simulink model "bms_controller"  (R2024b)
settings: Solver=FixedStepDiscrete  StartTime=0.0  StopTime=3600  FixedStep=0.1  RelTol=1e-3
undefined symbols (not defined in the file): DiscIntNeverNeededParam
libraries: simulink x6
settings Model: Creator=ferdi  LastModifiedBy=ferdi
settings OptimizationCC: DefaultParameterBehavior=Inlined  EnhancedBackFolding=on  PassReuseOutputArgsAs=Individual arguments  ZeroExternalMemoryAtStartup=off  ZeroInternalMemoryAtStartup=off  OptimizeBlockOrder=speed  DifferentSizesBufferReuse=on  OptimizationCustomize=off  EfficientTunableParamExpr=on
settings DebuggingCC: ParameterTunabilityLossMsg=error
settings HardwareCC: ProdBitPerPointer=32  ProdBitPerSizeT=32  ProdBitPerPtrDiffT=32  ProdLargestAtomicInteger=Long  ProdLargestAtomicFloat=Double  ProdWordSize=32  ProdHWDeviceType=ARM Compatible->ARM Cortex-M
settings SFSimCC: MATLABDynamicMemAlloc=off
settings RTWCC: Description=Embedded Coder  SystemTargetFile=ert.tlc  TemplateMakefile=ert_default_tmf
settings CodeAppCC: ForceParamTrailComments=on  IgnoreCustomStorageClasses=off  OperatorAnnotations=on  SimulinkDataObjDesc=on  SFDataObjDesc=on  InsertBlockDesc=on
settings ERTTargetCC: TargetLangStandard=C99 (ISO)  GenerateSampleERTMain=on  ERTCustomFileTemplate=example_file_process.tlc

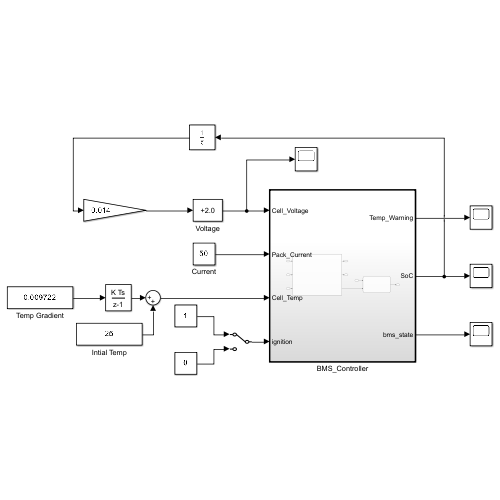
[thumbnail: Simulink's stored preview of the top-level diagram]
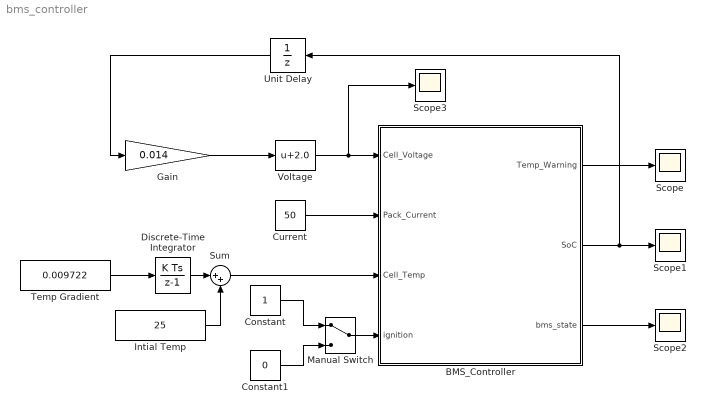
== system bms_controller ==
  BMS_Controller : Subsystem  TreatAsAtomicUnit=on  SystemSampleTime=0.1
  Constant : Constant  SampleTime=0.1
  Constant1 : Constant  Value=0  SampleTime=0.1
  Current : Constant  Value=50  SampleTime=0.1
  Discrete-Time Integrator : DiscreteIntegrator  SampleTime=0.1  ICPrevOutput=DiscIntNeverNeededParam  ICPrevScaledInput=DiscIntNeverNeededParam
  Gain : Gain  Gain=0.014
  Intial Temp : Constant  Value=25  SampleTime=0.1
  Manual Switch : ManualSwitch
  Scope{,1..3} (4 alike) : Scope
  Sum : Sum  Inputs=|++
  Temp Gradient : Constant  Value=0.009722  SampleTime=0.1
  Unit Delay : UnitDelay  InitialCondition=100  SampleTime=0.1  HasFrameUpgradeWarning=on
  Voltage : Bias  Bias=2.0  SaturateOnIntegerOverflow=off
  wires:
  Current/1 -> BMS_Controller/2(Pack_Current)
  Constant1/1 -> Manual Switch/2
  Constant/1 -> Manual Switch/1
  Manual Switch/1 -> BMS_Controller/4(ignition)
  BMS_Controller/1(Temp_Warning) -> Scope/1
  BMS_Controller/2(SoC) -> Unit Delay/1, Scope1/1
  BMS_Controller/3(bms_state) -> Scope2/1
  Temp Gradient/1 -> Discrete-Time Integrator/1
  Discrete-Time Integrator/1 -> Sum/1
  Intial Temp/1 -> Sum/2
  Sum/1 -> BMS_Controller/3(Cell_Temp)
  Voltage/1 -> Scope3/1, BMS_Controller/1(Cell_Voltage)
  Gain/1 -> Voltage/1
  Unit Delay/1 -> Gain/1

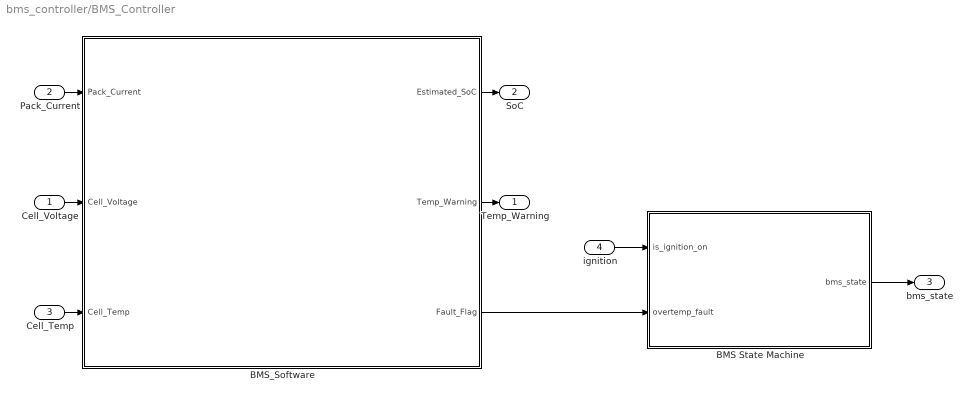
== system bms_controller/BMS_Controller ==
  Cell_Voltage : Inport
  Pack_Current : Inport  Port=2
  Cell_Temp : Inport  Port=3
  ignition : Inport  Port=4
  BMS State Machine : Stateflow chart  TreatAsAtomicUnit=on
  BMS_Software : Subsystem
  Temp_Warning : Outport
  SoC : Outport  Port=2
  bms_state : Outport  Port=3
  wires:
  BMS_Software/3(Fault_Flag) -> BMS State Machine/2(overtemp_fault)
  BMS_Software/2(Temp_Warning) -> Temp_Warning/1
  Pack_Current/1 -> BMS_Software/1(Pack_Current)
  Cell_Temp/1 -> BMS_Software/3(Cell_Temp)
  ignition/1 -> BMS State Machine/1(is_ignition_on)
  BMS_Software/1(Estimated_SoC) -> SoC/1
  BMS State Machine/1(bms_state) -> bms_state/1
  Cell_Voltage/1 -> BMS_Software/2(Cell_Voltage)

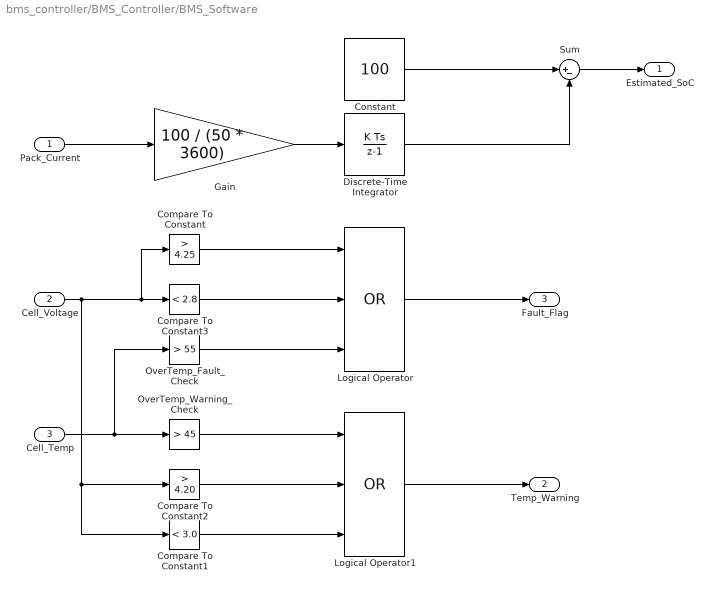
== system bms_controller/BMS_Controller/BMS_Software ==
  Pack_Current : Inport
  Cell_Voltage : Inport  Port=2
  Cell_Temp : Inport  Port=3
  Compare To Constant : simulink/Logic and Bit Operations/Compare To Constant  relop=>  const=4.25  OutDataTypeStr=boolean
  Compare To Constant1 : simulink/Logic and Bit Operations/Compare To Constant  relop=<  const=3.0  OutDataTypeStr=boolean
  Compare To Constant2 : simulink/Logic and Bit Operations/Compare To Constant  relop=>  const=4.20  OutDataTypeStr=boolean
  Compare To Constant3 : simulink/Logic and Bit Operations/Compare To Constant  relop=<  const=2.8  OutDataTypeStr=boolean
  Constant : Constant  Value=100
  Discrete-Time Integrator : DiscreteIntegrator  SampleTime=0.1  ICPrevOutput=DiscIntNeverNeededParam  ICPrevScaledInput=DiscIntNeverNeededParam
  Gain : Gain  Gain=100 / (50 * 3600)
  Logical Operator : Logic  Operator=OR  Inputs=3  AllPortsSameDT=off  OutDataTypeStr=boolean
  Logical Operator1 : Logic  Operator=OR  Inputs=3  AllPortsSameDT=off  OutDataTypeStr=boolean
  OverTemp_Fault_Check : simulink/Logic and Bit Operations/Compare To Constant  relop=>  const=55  OutDataTypeStr=boolean
  OverTemp_Warning_Check : simulink/Logic and Bit Operations/Compare To Constant  relop=>  const=45  OutDataTypeStr=boolean
  Sum : Sum  Inputs=|+-
  Estimated_SoC : Outport
  Temp_Warning : Outport  Port=2
  Fault_Flag : Outport  Port=3
  wires:
  Pack_Current/1 -> Gain/1
  Gain/1 -> Discrete-Time Integrator/1
  Sum/1 -> Estimated_SoC/1
  Constant/1 -> Sum/1
  Discrete-Time Integrator/1 -> Sum/2
  Cell_Temp/1 -> OverTemp_Fault_Check/1, OverTemp_Warning_Check/1
  OverTemp_Warning_Check/1 -> Logical Operator1/1
  OverTemp_Fault_Check/1 -> Logical Operator/3
  Cell_Voltage/1 -> Compare To Constant/1, Compare To Constant3/1, Compare To Constant1/1, Compare To Constant2/1
  Compare To Constant/1 -> Logical Operator/1
  Compare To Constant3/1 -> Logical Operator/2
  Logical Operator/1 -> Fault_Flag/1
  Compare To Constant2/1 -> Logical Operator1/2
  Compare To Constant1/1 -> Logical Operator1/3
  Logical Operator1/1 -> Temp_Warning/1

== stateflow chart bms_controller/BMS_Controller/BMS State Machine ==
  state Standby
    entry: bms_state = 0;
  state Drive
    entry: bms_state = 1;
  state Fault
    entry: bms_state = 2;
  (default) -> Standby
  Standby -> Fault [order 2] : [overtemp_fault == 1]
  Standby -> Drive [order 1] : [is_ignition_on == 1 && overtemp_fault == 0]
  Drive -> Standby [order 1] : [is_ignition_on == 0]
  Drive -> Fault [order 2] : [overtemp_fault == 1]
  data: is_ignition_on input; overtemp_fault input; bms_state output
